simulink model "Part9Step"  (R2024b)
settings: Solver=VariableStepAuto  StartTime=0.0  StopTime=10.0  RelTol=1e-3
values from neighbouring files (symbols this model uses):
  A = [0, 1; 0, -1/Tm]    [DesignPart567.m]    (also in DesignPart8.m; DesignPart9Sine.m; DesignPart9Step.m = [0, 1; 0, a22]; Init.m = [0, 1;0, -1/Tm])
  Ae = [Arho, zeros(size(Arho, 1), size(A, 1)); B*Crho, A]    [DesignPart9Sine.m]    (also in DesignPart9Step.m = [     Arho, zeros(size(Arho, 1), size(A, 1));      B*Crho, A; Init.m = [0  ,C; zeros(2, 1), A ])
  B = [0, km/(gbox.N*Tm)]'    [DesignPart567.m]    (also in DesignPart8.m; DesignPart9Sine.m; DesignPart9Step.m = [0, b2]'; Init.m = [0; drv.dcgain*mot.Kt/(gbox.N1*mot.Req*Jeq)])
  Be = [zeros(size(Arho, 1), 1); B]    [DesignPart9Sine.m]    (also in DesignPart9Step.m; Init.m = [0 ; B])
  C = [1, 0]    [DesignPart567.m]    (also in DesignPart8.m; DesignPart9Sine.m; DesignPart9Step.m; Init.m)
  Ce = [zeros(1, size(Arho, 1)), C]    [DesignPart9Sine.m]    (also in DesignPart9Step.m; Init.m = [0 C])
  Crho = [Cw, 0, 0]    [DesignPart9Sine.m]    (also in DesignPart9Step.m = 1)
  Cw1 = deg2rad * 1    [DesignPart9Step.m]
  Cw2 = deg2rad * 40    [DesignPart9Step.m]
  D = 0    [DesignPart567.m]    (also in DesignPart8.m; DesignPart9Sine.m; DesignPart9Step.m; Init.m)
  delta_est = 1/sqrt(2)    [DesignPart9Step.m]    (also in Init.m)
  K = real(K)    [DesignPart567.m]    (also in DesignPart8.m; DesignPart9Sine.m; DesignPart9Step.m = place(  A,   B, CtrlPoles); Init.m = acker(A,B,poles))
  L = real(L)    [DesignPart9Sine.m]    (also in DesignPart9Step.m = place(Ae', Ce', ObsvPoles)')
  wc = 2*pi*50    (= 314.159265359)    [DesignPart9Step.m]    (also in Init.m)
undefined symbols (not defined in the file or in its folder): drv, sens
settings Model: Creator=Banaan  LastModifiedBy=Banaan

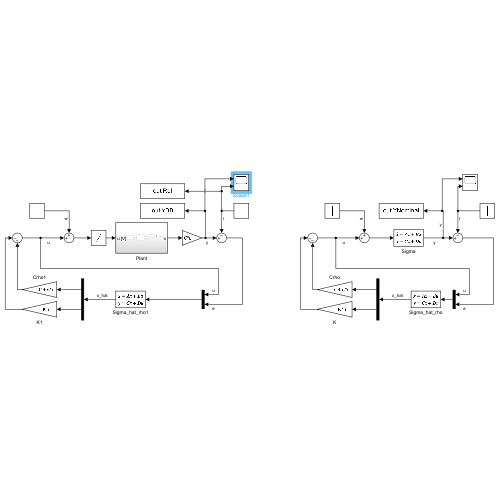
[thumbnail: Simulink's stored preview of the top-level diagram]
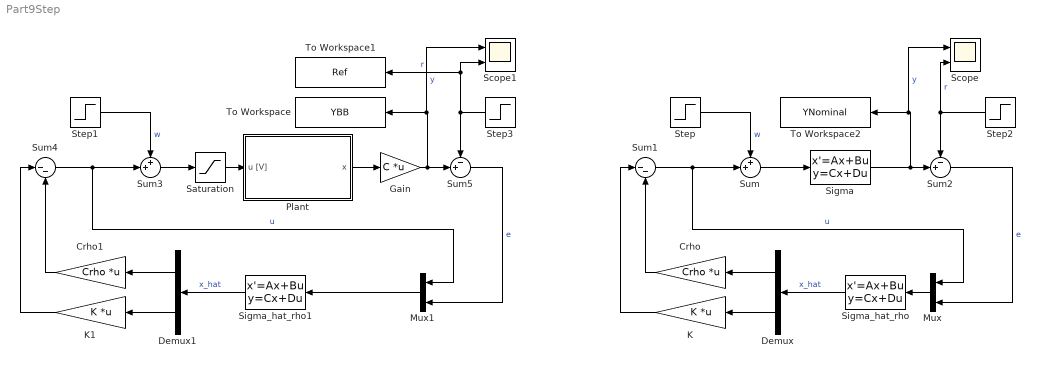
== system Part9Step ==
  Crho : Gain  Gain=Crho  Multiplication=Matrix(K*u)
  Crho1 : Gain  Gain=Crho  Multiplication=Matrix(K*u)
  Demux : Demux  Outputs=2
  Demux1 : Demux  Outputs=2
  Gain : Gain  Gain=C  Multiplication=Matrix(K*u)
  K : Gain  Gain=K  Multiplication=Matrix(K*u)
  K1 : Gain  Gain=K  Multiplication=Matrix(K*u)
  Mux : Mux  Inputs=2
  Mux1 : Mux  Inputs=2
  Plant : Subsystem
  Saturation : Saturate  UpperLimit=10  LowerLimit=-10
  Scope : Scope  NumInputPorts=2
  Scope1 : Scope  NumInputPorts=2
  Sigma : StateSpace  A=A  B=B  C=C  D=D  InitialCondition=rand(2, 1)
  Sigma_hat_rho : StateSpace  A=Ae - L*Ce  B=[Be, L]  C=eye(4)  D=zeros(4, 2)  InitialCondition=rand(4, 1)
  Sigma_hat_rho1 : StateSpace  A=Ae - L*Ce  B=[Be, L]  C=eye(4)  D=zeros(4, 2)  InitialCondition=rand(4, 1)
  Step : Step  After=Cw1  SampleTime=0
  Step1 : Step  After=Cw1  SampleTime=0
  Step2 : Step  After=Cw2  SampleTime=0
  Step3 : Step  After=Cw2  SampleTime=0
  Sum : Sum  Inputs=++|
  Sum1 : Sum  Inputs=|--
  Sum2 : Sum  Inputs=-+|
  Sum3 : Sum  Inputs=++|
  Sum4 : Sum  Inputs=|--
  Sum5 : Sum  Inputs=-+|
  To Workspace : ToWorkspace  VariableName=YBB  SaveFormat=Timeseries  SampleTime=-1
  To Workspace1 : ToWorkspace  VariableName=Ref  SaveFormat=Timeseries  SampleTime=-1
  To Workspace2 : ToWorkspace  VariableName=YNominal  SaveFormat=Timeseries  SampleTime=-1
  wires:
  Sum/1 -> Sigma/1
  Demux/2 -> K/1
  Sum2/1 -> Mux/2  "e"
  Demux1/1 -> Crho1/1
  Sum4/1 -> Mux1/1, Sum3/2  "u"
  Saturation/1 -> Plant/1(u [V])
  K1/1 -> Sum4/1
  Sigma/1 -> Scope/1, To Workspace2/1, Sum2/2  "y"
  Mux/1 -> Sigma_hat_rho/1
  Step/1 -> Sum/1  "w"
  Sum1/1 -> Sum/2, Mux/1  "u"
  Sigma_hat_rho1/1 -> Demux1/1  "x_hat"
  K/1 -> Sum1/1
  Demux1/2 -> K1/1
  Gain/1 -> Scope1/1, To Workspace/1, Sum5/2  "y"
  Sigma_hat_rho/1 -> Demux/1  "x_hat"
  Sum5/1 -> Mux1/2  "e"
  Sum3/1 -> Saturation/1
  Crho1/1 -> Sum4/2
  Step1/1 -> Sum3/1  "w"
  Step2/1 -> Sum2/1, Scope/2  "r"
  Plant/1(x) -> Gain/1
  Step3/1 -> Sum5/1, Scope1/2, To Workspace1/1  "r"
  Demux/1 -> Crho/1
  Crho/1 -> Sum1/2
  Mux1/1 -> Sigma_hat_rho1/1

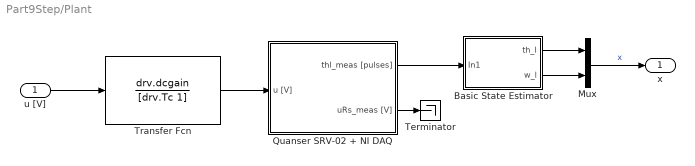
== system Part9Step/Plant ==
  u [V] : Inport
  Basic State Estimator : Subsystem
  Mux : Mux  Inputs=2
  Quanser SRV-02 + NI DAQ : Subsystem  mask(Quanser SRV-02 (with inertial load) + NI DAQ){Ts=0.001, fricType=Coulomb + viscous}
      mask prompts: Ts "NI DAQ Sample Time:"; fricType "Friction model"
      mask help: Quanser SRV-02 (with inertial load) + NI DAQ model.
      mask init:
      | %%  Sensors data
      | 
      | %   shunt resistor
      | sens.curr.Rs = 0.5;                         %   resistance [Ohm]   
      | sens.curr.uRs_std = 0.01;                   %   voltage noise standard dev [V]                           
      | sens.curr.uRs_var = sens.curr.uRs_std^2;	%   voltage noise variance [V^2]
      | 
      | %   Hewlett-Packard HEDS-5540#A06 optical encoder
      | sens.enc.ppr = 500*4;                       %   pulses per rotation
      | sens.enc.pulse2deg = 360/sens.enc.ppr;      %   [pulses] -> [deg]
      | sens.enc.pulse2rad = 2*pi/sens.enc.ppr;     %   [pulses] -> [rad]
      | sens.enc.deg2pulse = sens.enc.ppr/360;      %   [deg] -> [pulses]
      | sens.enc.rad2pulse = sens.enc.ppr/2/pi;     %   [rad] -> [pulses]
      | 
      | 
      | %%  Data acquisition board (daq) data
      | 
      | %   NI PCI-6221 DAC data
      | daq.dac.bits = 16;                                  %   resolution (bits)
      | daq.dac.fs   = 10;                                  %   full scale 
      | daq.dac.q    = 2*daq.dac.fs/(2^daq.dac.bits-1);     %	quantization
      | 
      | %   NI PCI-6221 ADC data
      | daq.adc.bits = 16;                                  %   resolution (bits)
      | daq.adc.fs   = 10;                                  %   full scale (as set in SLDRT Analog Input block)
      | daq.adc.q    = 2*daq.adc.fs/(2^daq.adc.bits-1);     %   quantization
      mask Help:
      | Riccardo Antonello (antonello@dei.unipd.it)
      | 
      | April 24, 2020
      | 
      | Dept. of Information Engineering, University of Padova
      mask TypeOptions fricType: Coulomb + viscous | Karnopp
  Terminator : Terminator
  Transfer Fcn : TransferFcn  Numerator=drv.dcgain  Denominator=[drv.Tc 1]
  x : Outport
  wires:
  u [V]/1 -> Transfer Fcn/1
  Basic State Estimator/1(th_l) -> Mux/1
  Basic State Estimator/2(w_l) -> Mux/2
  Quanser SRV-02 + NI DAQ/1(thl_meas [pulses]) -> Basic State Estimator/1(In1)
  Mux/1 -> x/1  "x"
  Quanser SRV-02 + NI DAQ/2(uRs_meas [V]) -> Terminator/1
  Transfer Fcn/1 -> Quanser SRV-02 + NI DAQ/1(u [V])

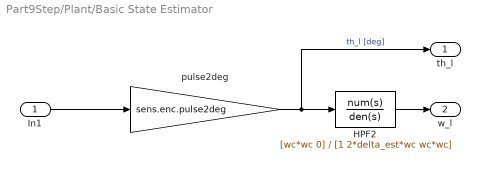
== system Part9Step/Plant/Basic State Estimator ==
  In1 : Inport
  HPF2 : TransferFcn  Numerator=[wc*wc 0]  Denominator=[1 2*delta_est*wc wc*wc]
  pulse2deg : Gain  Gain=sens.enc.pulse2deg
  th_l : Outport
  w_l : Outport  Port=2
  wires:
  pulse2deg/1 -> th_l/1, HPF2/1  "th_l [deg]"
  In1/1 -> pulse2deg/1
  HPF2/1 -> w_l/1

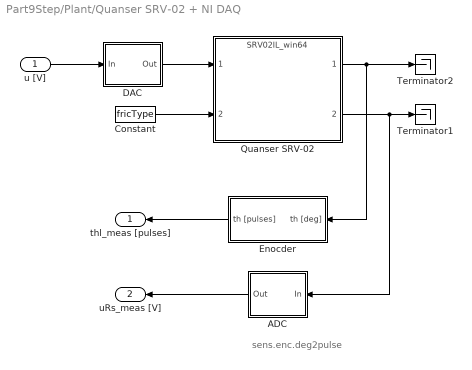
== system Part9Step/Plant/Quanser SRV-02 + NI DAQ ==
  note: sens.enc.deg2pulse
  u [V] : Inport
  ADC : Subsystem
  Constant : Constant  Value=fricType
  DAC : Subsystem
  Enocder : Subsystem
  Quanser SRV-02 : ModelReference  ModelNameDialog=SRV02IL_win64.slxp  ModelReferenceVersion=1.44  CopyOfModelProtected=on
  Terminator1 : Terminator
  Terminator2 : Terminator
  thl_meas [pulses] : Outport
  uRs_meas [V] : Outport  Port=2
  wires:
  Enocder/1(th [pulses]) -> thl_meas [pulses]/1
  ADC/1(Out) -> uRs_meas [V]/1
  DAC/1(Out) -> Quanser SRV-02/1
  Quanser SRV-02/2 -> ADC/1(In), Terminator1/1
  u [V]/1 -> DAC/1(In)
  Quanser SRV-02/1 -> Enocder/1(th [deg]), Terminator2/1
  Constant/1 -> Quanser SRV-02/2

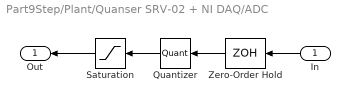
== system Part9Step/Plant/Quanser SRV-02 + NI DAQ/ADC ==
  In : Inport
  Quantizer : Quantizer  QuantizationInterval=daq.adc.q
  Saturation : Saturate  UpperLimit=daq.adc.fs  LowerLimit=-daq.adc.fs
  Zero-Order Hold : ZeroOrderHold  SampleTime=Ts
  Out : Outport
  wires:
  Saturation/1 -> Out/1
  In/1 -> Zero-Order Hold/1
  Quantizer/1 -> Saturation/1
  Zero-Order Hold/1 -> Quantizer/1

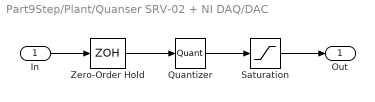
== system Part9Step/Plant/Quanser SRV-02 + NI DAQ/DAC ==
  In : Inport
  Quantizer : Quantizer  QuantizationInterval=daq.dac.q
  Saturation : Saturate  UpperLimit=daq.dac.fs  LowerLimit=-daq.dac.fs
  Zero-Order Hold : ZeroOrderHold  SampleTime=Ts
  Out : Outport
  wires:
  Quantizer/1 -> Saturation/1
  In/1 -> Zero-Order Hold/1
  Zero-Order Hold/1 -> Quantizer/1
  Saturation/1 -> Out/1

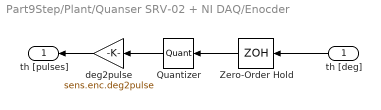
== system Part9Step/Plant/Quanser SRV-02 + NI DAQ/Enocder ==
  th [deg] : Inport
  Quantizer : Quantizer  QuantizationInterval=sens.enc.pulse2deg
  Zero-Order Hold : ZeroOrderHold  SampleTime=Ts
  deg2pulse : Gain  Gain=sens.enc.deg2pulse
  th [pulses] : Outport
  wires:
  Quantizer/1 -> deg2pulse/1
  th [deg]/1 -> Zero-Order Hold/1
  Zero-Order Hold/1 -> Quantizer/1
  deg2pulse/1 -> th [pulses]/1
